simulink model "supervisor_big_little"  (R2016a)
settings: Solver=FixedStepDiscrete  StartTime=0.0  StopTime=10.0  FixedStep=0.1  RelTol=1e-3
settings Model: Creator=kmoaz_000  LastModifiedBy=kmoaz_000
settings SolverCC: AutoInsertRateTranBlk=on
settings DataIOCC: LimitDataPoints=on
settings DebuggingCC: AllowSymbolicDim=off
settings ConfigComp: CovModelRefEnable=Off  CovSFcnEnable=off

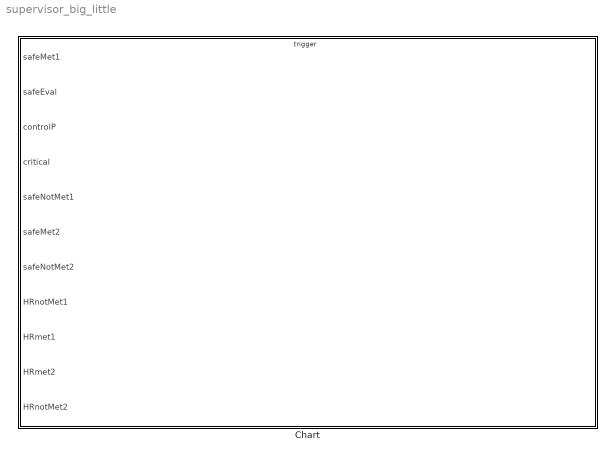
== system supervisor_big_little ==
  Chart : Stateflow chart  TreatAsAtomicUnit=on

== stateflow chart supervisor_big_little/Chart ==
  state SafeEval_QOSmet2
  state SafeEval_QOSnotMet2
  state QOSMet1_SafeEval2
  state QOSnotMet1_SafeEval2
  state SafeEva_SafeEval2l
  state QOSMet1_QOSMet2
  state SwitchGains
  state PowerCap
  state dangerPower
  state QOSMet1_QOSnotMet2
  state QOSnotMet1_QOSmet2
  state QOSnotMet1_QOSnotMet2
  SafeEval_QOSmet2 -> SafeEval_QOSmet2 [order 1] : decreaseP2{Decrease_P2()}
  SafeEval_QOSmet2 -> QOSMet1_QOSMet2 [order 2] : [safeMet1]
  SafeEval_QOSmet2 -> QOSnotMet1_QOSmet2 [order 3] : [HRnotMet1]
  SafeEva_SafeEval2l -> SafeEval_QOSmet2 [order 4] : [safeMet2]
  SafeEval_QOSnotMet2 -> SafeEval_QOSmet2 [order 4] : [HRmet2]
  SafeEval_QOSmet2 -> SafeEval_QOSnotMet2 [order 4] : [HRnotMet2]
  SafeEval_QOSnotMet2 -> QOSnotMet1_QOSnotMet2 [order 3] : [HRnotMet1]
  SafeEval_QOSnotMet2 -> SafeEval_QOSnotMet2 [order 2] : increaseP2{Increase_P2()}
  SafeEva_SafeEval2l -> SafeEval_QOSnotMet2 [order 3] : [safeNotMet2]
  SafeEval_QOSnotMet2 -> QOSMet1_QOSnotMet2 [order 1] : [HRmet1]
  QOSMet1_SafeEval2 -> QOSMet1_SafeEval2 [order 4] : decreaseP1{Decrease_P1()}
  QOSMet1_SafeEval2 -> QOSMet1_QOSMet2 [order 1]
  SafeEva_SafeEval2l -> QOSMet1_SafeEval2 [order 2] : [safeMet1]
  QOSMet1_SafeEval2 -> QOSMet1_QOSnotMet2 [order 2] : [HRnotMet2]
  QOSMet1_SafeEval2 -> QOSnotMet1_SafeEval2 [order 3] : [HRnotMet1]
  QOSnotMet1_SafeEval2 -> QOSMet1_SafeEval2 [order 4] : [HRmet1]
  QOSnotMet1_SafeEval2 -> QOSnotMet1_QOSnotMet2 [order 2] : [HRnotMet2]
  QOSnotMet1_SafeEval2 -> QOSnotMet1_QOSmet2 [order 1] : [HRmet2]
  SafeEva_SafeEval2l -> QOSnotMet1_SafeEval2 [order 1] : [safeNotMet1]
  QOSnotMet1_SafeEval2 -> QOSnotMet1_SafeEval2 [order 3] : increaseP1{Increase_P1()}
  (default) -> QOSMet1_QOSMet2
  SwitchGains -> SafeEva_SafeEval2l [order 2] : [safeEval]
  QOSMet1_QOSnotMet2 -> QOSMet1_QOSnotMet2 [order 3] : decreaseP1{Decrease_P1}
  QOSMet1_QOSMet2 -> QOSMet1_QOSMet2 [order 4] : decreaseP2{Decrease_P2()}
  QOSMet1_QOSnotMet2 -> QOSMet1_QOSnotMet2 [order 5] : increaseP2{Increase_P2}
  QOSMet1_QOSnotMet2 -> QOSMet1_QOSMet2 [order 1] : [HRmet2]
  PowerCap -> dangerPower [order 1] : [critical]
  QOSnotMet1_QOSmet2 -> QOSMet1_QOSMet2 [order 1] : [HRmet1]
  SwitchGains -> PowerCap [order 1] : [controlP]
  QOSMet1_QOSMet2 -> SwitchGains [order 2] : [critical]
  QOSMet1_QOSMet2 -> QOSMet1_QOSMet2 [order 1] : decreaseP1{Decrease_P1()}
  QOSMet1_QOSMet2 -> QOSnotMet1_QOSmet2 [order 5] : [HRnotMet1]
  QOSMet1_QOSMet2 -> QOSMet1_QOSnotMet2 [order 3] : [HRnotMet2]
  dangerPower -> PowerCap [order 1] : [safeP]
  PowerCap -> SwitchGains [order 2] : [safeP]
  QOSMet1_QOSnotMet2 -> SwitchGains [order 2] : [critical]
  QOSnotMet1_QOSmet2 -> SwitchGains [order 2] : [critical]
  QOSMet1_QOSnotMet2 -> QOSnotMet1_QOSnotMet2 [order 4] : [HRnotMet1]
  QOSnotMet1_QOSnotMet2 -> SwitchGains [order 1] : [critical]
  PowerCap -> PowerCap [order 3] : decreaseCritical{DecreaseCriticalP1(),DecreaseCriticalP2()}
  dangerPower -> dangerPower [order 2] : decreaseCritical{DecreaseCriticalP1(),DecreaseCriticalP2()}
  QOSnotMet1_QOSnotMet2 -> QOSMet1_QOSnotMet2 [order 2] : [HRmet1]
  QOSnotMet1_QOSmet2 -> QOSnotMet1_QOSmet2 [order 4] : decreaseP2{Decrease_P2()}
  QOSnotMet1_QOSnotMet2 -> QOSnotMet1_QOSmet2 [order 3] : [HRmet2]
  QOSnotMet1_QOSmet2 -> QOSnotMet1_QOSnotMet2 [order 3] : [HRnotMet2]
  QOSnotMet1_QOSmet2 -> QOSnotMet1_QOSmet2 [order 5] : increaseP1{Increase_P1()}
  QOSnotMet1_QOSnotMet2 -> QOSnotMet1_QOSnotMet2 [order 5] : increaseP2{Increase_P2()}
  QOSnotMet1_QOSnotMet2 -> QOSnotMet1_QOSnotMet2 [order 4] : increaseP1{Increase_P1()}
  data: safeMet1 input; safeEval input; controlP input; critical input; safeNotMet1 input; safeMet2 input; safeNotMet2 input; HRnotMet1 input; HRmet1 input; HRmet2 input; HRnotMet2 input
  events: decreaseP2 input RISING_EDGE_EVENT; decrease_P2 input RISING_EDGE_EVENT; event1 input RISING_EDGE_EVENT; event2 input RISING_EDGE_EVENT; safeP input RISING_EDGE_EVENT; decreaseCritical input RISING_EDGE_EVENT; decreaseP1 input RISING_EDGE_EVENT; Met1_NotMet2 input RISING_EDGE_EVENT; increaseP2 input RISING_EDGE_EVENT; increaseP1 input RISING_EDGE_EVENT
  function DecreaseCriticalP1:
    | function DecreaseCriticalP1
  function DecreaseCriticalP2:
    | function DecreaseCriticalP2
  function Decrease_P1:
    | function Decrease_P1  %#codegen
    | y = 'Im gonna change a parametter'
  function Decrease_P2:
    | function Decrease_P2
  function Increase_P1:
    | function Increase_P1
  function Increase_P2:
    | function Increase_P2
